simulink model "SF015A_WhlImbRejctn"  (R2013b)
settings: Solver=FixedStepDiscrete  SolverMode=SingleTasking  StartTime=0.0  StopTime=1  FixedStep=0.002  RelTol=1e-3
undefined symbols (not defined in the file): ACTIVBANDMAX_ULS_U32, ADAPVFILMAX_ULS_F32, ADJOUTPMAX_ULS_F32, ARCHGLBPRM_180OVERPI_ULS_F32, ARCHGLBPRM_2MILLISEC_SEC_F32, ARCHGLBPRM_2PI_ULS_F32, ARCHGLBPRM_FLOATZEROTHD_ULS_F32, ARCHGLBPRM_PI_ULS_F32, ARCHGLBPRM_PIOVER180_ULS_F32, ARCHGLBPRM_PIOVER2_ULS_F32, CALMINSPERCOUNT_ULS_F32, Cntr, DURATIONDISABLE_CNT_U16, FILTWHLSPDMAX_MOTRADPERSEC_F32, FRQMIN_ULS_F32, MICROSECTOMILLISEC_ULS_F32, MINSTOMILLISEC_ULS_F32, NINETY_ULS_F32, NODEBSTEP_CNT_U16, NROFDLY_CNT_U08, NtcSts1, NvmGetErrSts1, ONEHALF_ULS_F32, ONEHUNDRED_ULS_F32, ONEOVRTHREE_ULS_F32, ONEOVRTWENTY_ULS_F32, ONETHOUSAND_ULS_F32, PEAKMAX_ULS_F32, PEAKMIN_ULS_F32, PHAADJMAX_ULS_F32, PITIMESSAMPLETIME_ULS_F32, SigQlfr1, STOREDMINSPERCOUNT_ULS_F32, Sts, SysSt1, TWO_ULS_F32, TWOOVRTHREE_ULS_F32, UGRFILMAX_ULS_F32, WhlImbRejctnAdpvFac, WhlImbRejctnAutScaEna, WhlImbRejctnAutScaTar, WhlImbRejctnCurrMgnSlewPerLoop, WhlImbRejctnDcTrendFltRcvryDly, WhlImbRejctnDcTrendFltRcvryNegStep, WhlImbRejctnDcTrendFltRcvryPosStep, WhlImbRejctnDcTrendFltRcvryThd, WhlImbRejctnDcTrendTh2Tq, WhlImbRejctnDcTrendThTq, WhlImbRejctnDcTrendTi2Sec, WhlImbRejctnDcTrendTiSec, WhlImbRejctnEnaSlewPerLoop, WhlImbRejctnFctEna, WhlImbRejctnFltNtc, WhlImbRejctnFrqDiagcAmpThd, WhlImbRejctnFrqDiagcEna, WhlImbRejctnFrqDiagcFltRcvryDly, WhlImbRejctnFrqDiagcFltRcvryNegStep, WhlImbRejctnFrqDiagcFltRcvryPosStep, WhlImbRejctnFrqDiagcFltRcvryThd, WhlImbRejctnFrqDiagcThd ... (+30)
libraries: FixdToFloat x32, simulink x26, NxtrLim x25, Fil x20, NxtrAbslt x9, NxtrMath x7, NxtrMax x6, NxtrMin x4, NxtrNvM x2, FloatToFixd x2, LnrIntrpn x2, NxtrSign x1
(part 5 of 14)

== system SF015A_WhlImbRejctn/WhlImbRejctn/WhlImbRejctnPer2/Flt Recovery- WhlSpdCorr Diag/Update Fault Status ==
  Structvar : Inport
  Status : Inport  Port=2
  Bus Assignment : BusAssignment  AssignedSignals=Cntr,Sts
  Bus Selector : BusSelector  OutputSignals=Cntr,Sts,Thd,NegStep,PosStep
  Compare To Zero : simulink/Logic and Bit Operations/Compare To Zero  relop=<=  OutDataTypeStr=boolean
  Constant : Constant  Value=0  OutDataTypeStr=single
  CopyRight2 : Subsystem  Description=|  mask(Copyright Information){none=on}
      | Copyright info block.                                               
      |                                                                     
      | Place copyright information at the top of every subsystem in design.
      mask prompts: none "No parameters"
      mask help: Place copyright information at the top of every subsystem in design.
      mask Display:
      | NxtrConf = 'Nexteer Confidential';
      | 
      | sys = bdroot; %handle for the current model ("system")
      | first = get_param(sys,'Created');
      | first = first(end-3:end);  %year is last four digits
      | 
      | last = get_param(sys,'LastModifiedDate');
      | if isempty(last)
      |     last = datestr(now,'yyyy');
      | else
      |     last = last(end-3:end);
      | end
      | 
      | if strcmp(first,last)
      |     fprintf('%s -- Copyright %s Nexteer',NxtrConf,first)
      | else
      |     fprintf('%s -- %s%s- %s Nexteer',NxtrConf,char(169),first,last)
      | end
  Enumerated Constant : simulink/Sources/Enumerated Constant  OutDataTypeStr=Enum: SigQlfr1  Value=SigQlfr1.SIGQLFR_FAILD  SampleTime=inf
  Enumerated Constant1 : simulink/Sources/Enumerated Constant  OutDataTypeStr=Enum: SigQlfr1  Value=SigQlfr1.SIGQLFR_PASSD  SampleTime=inf
  If : If  IfExpression=u1
  If1 : If  NumInputs=2  IfExpression=u1  ElseIfExpressions=u2  ShowElse=off
  Merge : Merge
  Relational Operator : RelationalOperator  OutDataTypeStr=boolean
  Terminator : Terminator
  Towards Failed : Subsystem  TreatAsAtomicUnit=on
  Towards Passed : Subsystem  TreatAsAtomicUnit=on
  Update to Failed : Subsystem  TreatAsAtomicUnit=on
  Update to Passed : Subsystem  TreatAsAtomicUnit=on
  counter : Merge
  Structvar_out : Outport
  wires:
  Structvar/1 -> Bus Assignment/1, Bus Selector/1
  Status/1 -> If/1
  If/1 -> Towards Failed/Action
  If/2 -> Towards Passed/Action
  [PosStep] -> Towards Failed/1(PosStep)
  [NegStep] -> Towards Passed/1(NegStep)
  Towards Failed/1(Out1) -> counter/1
  Towards Passed/1(Out1) -> counter/2
  [Cnt] -> Towards Failed/2(Cnt)
  [Thd] -> Towards Failed/3(Thd)
  Constant/1 -> Towards Passed/3(Thd)
  counter/1 -> [Cnt_update], Compare To Zero/1, Relational Operator/1
  Relational Operator/1 -> If1/1
  If1/1 -> Update to Failed/Action
  If1/2 -> Update to Passed/Action
  Compare To Zero/1 -> If1/2
  Enumerated Constant1/1 -> Update to Passed/1(In1)
  Update to Failed/1(Out1) -> Merge/1
  Update to Passed/1(Out1) -> Merge/2
  Enumerated Constant/1 -> Update to Failed/1(In1)
  Bus Assignment/1 -> Structvar_out/1
  Merge/1 -> [Sts_update]
  Bus Selector/1 -> [Cnt]  "<Cntr>"
  Bus Selector/3 -> [Thd]  "<Thd>"
  Bus Selector/4 -> [NegStep]  "<NegStep>"
  Bus Selector/5 -> [PosStep]  "<PosStep>"
  [Cnt_update] -> Bus Assignment/2
  [Sts_update] -> Bus Assignment/3
  [Cnt] -> Towards Passed/2(Cnt)
  [Thd] -> Relational Operator/2
  Bus Selector/2 -> Terminator/1  "<Sts>"

== system SF015A_WhlImbRejctn/WhlImbRejctn/WhlImbRejctnPer2/WIR Low Speed Diagnostics/CopyRight2 ==

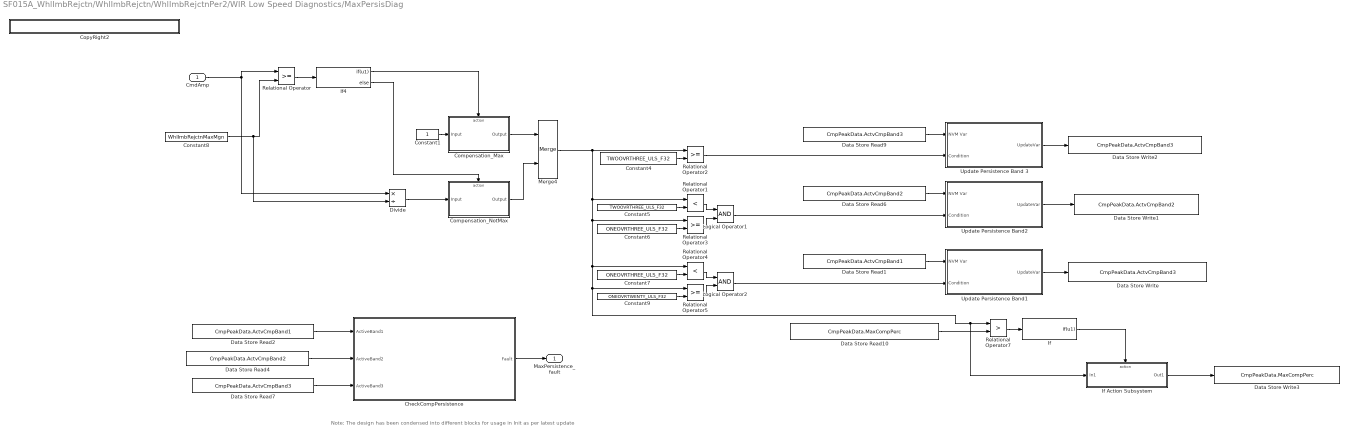
== system SF015A_WhlImbRejctn/WhlImbRejctn/WhlImbRejctnPer2/WIR Low Speed Diagnostics/MaxPersisDiag ==
  note: Note: The design has been condensed into different blocks for usage in Init as per latest update
  CmdAmp : Inport
  CheckCompPersistence : Subsystem
  Compensation_Max : Subsystem  RequirementInfo={} %GIDa_1bfe11f8_96f1_4e8d_9095_de3761426c03  TreatAsAtomicUnit=on
  Compensation_NotMax : Subsystem  RequirementInfo={} %GIDa_7b4c2964_e6f7_461b_b06a_d505129df27a  TreatAsAtomicUnit=on
  Constant1 : Constant  OutDataTypeStr=single
  Constant4 : Constant  Value=TWOOVRTHREE_ULS_F32
  Constant5 : Constant  Value=TWOOVRTHREE_ULS_F32
  Constant6 : Constant  Value=ONEOVRTHREE_ULS_F32
  Constant7 : Constant  Value=ONEOVRTHREE_ULS_F32
  Constant8 : Constant  Value=WhlImbRejctnMaxMgn
  Constant9 : Constant  Value=ONEOVRTWENTY_ULS_F32
  CopyRight2 : Subsystem  Description=|  mask(Copyright Information){none=on}
      | Copyright info block.                                               
      |                                                                     
      | Place copyright information at the top of every subsystem in design.
      mask prompts: none "No parameters"
      mask help: Place copyright information at the top of every subsystem in design.
      mask Display:
      | NxtrConf = 'Nexteer Confidential';
      | 
      | sys = bdroot; %handle for the current model ("system")
      | first = get_param(sys,'Created');
      | first = first(end-3:end);  %year is last four digits
      | 
      | last = get_param(sys,'LastModifiedDate');
      | if isempty(last)
      |     last = datestr(now,'yyyy');
      | else
      |     last = last(end-3:end);
      | end
      | 
      | if strcmp(first,last)
      |     fprintf('%s -- Copyright %s Nexteer',NxtrConf,first)
      | else
      |     fprintf('%s -- %s%s- %s Nexteer',NxtrConf,char(169),first,last)
      | end
  Data Store Read1 : DataStoreRead  Priority=1  DataStoreName=CmpPeakData  DataStoreElements=CmpPeakData.ActvCmpBand1
      settings: AttributesFormatString=Priority=%<Priority>
  Data Store Read10 : DataStoreRead  DataStoreName=CmpPeakData  DataStoreElements=CmpPeakData.MaxCompPerc
  Data Store Read2 : DataStoreRead  Priority=3  DataStoreName=CmpPeakData  DataStoreElements=CmpPeakData.ActvCmpBand1
      settings: AttributesFormatString=Priority=%<Priority>
  Data Store Read4 : DataStoreRead  Priority=3  DataStoreName=CmpPeakData  DataStoreElements=CmpPeakData.ActvCmpBand2
      settings: AttributesFormatString=Priority=%<Priority>
  Data Store Read6 : DataStoreRead  Priority=1  DataStoreName=CmpPeakData  DataStoreElements=CmpPeakData.ActvCmpBand2
      settings: AttributesFormatString=Priority=%<Priority>
  Data Store Read7 : DataStoreRead  Priority=3  DataStoreName=CmpPeakData  DataStoreElements=CmpPeakData.ActvCmpBand3
      settings: AttributesFormatString=Priority=%<Priority>
  Data Store Read9 : DataStoreRead  Priority=1  DataStoreName=CmpPeakData  DataStoreElements=CmpPeakData.ActvCmpBand3
      settings: AttributesFormatString=Priority=%<Priority>
  Data Store Write : DataStoreWrite  Priority=2  DataStoreName=CmpPeakData  DataStoreElements=CmpPeakData.ActvCmpBand3
      settings: AttributesFormatString=Priority=%<Priority>
  Data Store Write1 : DataStoreWrite  Priority=2  DataStoreName=CmpPeakData  DataStoreElements=CmpPeakData.ActvCmpBand2
      settings: AttributesFormatString=Priority=%<Priority>
  Data Store Write2 : DataStoreWrite  Priority=2  DataStoreName=CmpPeakData  DataStoreElements=CmpPeakData.ActvCmpBand3
      settings: AttributesFormatString=Priority=%<Priority>
  Data Store Write3 : DataStoreWrite  DataStoreName=CmpPeakData  DataStoreElements=CmpPeakData.MaxCompPerc
  Divide : Product  Inputs=*/
  If : If  IfExpression=u1  ShowElse=off
  If Action Subsystem : Subsystem  TreatAsAtomicUnit=on
  If4 : If  IfExpression=u1
  Logical Operator1 : Logic  AllPortsSameDT=off  OutDataTypeStr=boolean
  Logical Operator2 : Logic  AllPortsSameDT=off  OutDataTypeStr=boolean
  Merge4 : Merge
  Relational Operator{,2..3,5} (4 alike) : RelationalOperator  OutDataTypeStr=boolean
  Relational Operator1 : RelationalOperator  Operator=<  OutDataTypeStr=boolean
  Relational Operator4 : RelationalOperator  Operator=<  OutDataTypeStr=boolean
  Relational Operator7 : RelationalOperator  Operator=>  OutDataTypeStr=boolean
  Update Persistence Band 3 : Subsystem
  Update Persistence Band1 : Subsystem
  Update Persistence Band2 : Subsystem
  MaxPersistence_fault : Outport
  wires:
  CmdAmp/1 -> Relational Operator/1, Divide/1
  Constant8/1 -> Divide/2, Relational Operator/2
  Merge4/1 -> If Action Subsystem/1(In1), Relational Operator7/1, Relational Operator5/1, Relational Operator4/1, Relational Operator3/1, Relational Operator1/1, Relational Operator2/1
  Constant6/1 -> Relational Operator3/2
  Constant4/1 -> Relational Operator2/2
  Constant5/1 -> Relational Operator1/2
  Constant9/1 -> Relational Operator5/2
  Constant7/1 -> Relational Operator4/2
  Relational Operator3/1 -> Logical Operator1/2
  Relational Operator1/1 -> Logical Operator1/1
  Relational Operator4/1 -> Logical Operator2/1
  Relational Operator5/1 -> Logical Operator2/2
  Logical Operator1/1 -> Update Persistence Band2/2(Condition)
  Relational Operator7/1 -> If/1
  Data Store Read10/1 -> Relational Operator7/2
  If/1 -> If Action Subsystem/Action
  If Action Subsystem/1(Out1) -> Data Store Write3/1
  Relational Operator/1 -> If4/1
  Compensation_Max/1(Output) -> Merge4/1
  If4/1 -> Compensation_Max/Action
  Constant1/1 -> Compensation_Max/1(Input)
  Compensation_NotMax/1(Output) -> Merge4/2
  If4/2 -> Compensation_NotMax/Action
  Divide/1 -> Compensation_NotMax/1(Input)
  Data Store Read9/1 -> Update Persistence Band 3/1(NVM Var)
  Update Persistence Band 3/1(UpdateVar) -> Data Store Write2/1
  Relational Operator2/1 -> Update Persistence Band 3/2(Condition)
  Data Store Read6/1 -> Update Persistence Band2/1(NVM Var)
  Update Persistence Band2/1(UpdateVar) -> Data Store Write1/1
  Logical Operator2/1 -> Update Persistence Band1/2(Condition)
  Data Store Read1/1 -> Update Persistence Band1/1(NVM Var)
  Update Persistence Band1/1(UpdateVar) -> Data Store Write/1
  Data Store Read2/1 -> CheckCompPersistence/1(ActiveBand1)
  Data Store Read4/1 -> CheckCompPersistence/2(ActiveBand2)
  Data Store Read7/1 -> CheckCompPersistence/3(ActiveBand3)
  CheckCompPersistence/1(Fault) -> MaxPersistence_fault/1

== system SF015A_WhlImbRejctn/WhlImbRejctn/WhlImbRejctnInit1/Check NVM Data/CheckCompPersistence/CopyRight2 ==

== system SF015A_WhlImbRejctn/WhlImbRejctn/WhlImbRejctnInit1/Check NVM Data/CheckCompPersistence/NoFault ==
  Input : Inport
  Action Port : ActionPort  ActionType=else
  CopyRight2 : Subsystem  Description=|  mask(Copyright Information){none=on}
      | Copyright info block.                                               
      |                                                                     
      | Place copyright information at the top of every subsystem in design.
      mask prompts: none "No parameters"
      mask help: Place copyright information at the top of every subsystem in design.
      mask Display:
      | NxtrConf = 'Nexteer Confidential';
      | 
      | sys = bdroot; %handle for the current model ("system")
      | first = get_param(sys,'Created');
      | if(isempty(first))
      |     first = datestr(now,'yyyy');
      | else
      |     first = first(end-3:end);  %year is last four digits
      | end
      | 
      | last = get_param(sys,'LastModifiedDate');
      | if isempty(last)
      |     last = datestr(now,'yyyy');
      | else
      |     last = last(end-3:end);
      | end
      | 
      | if strcmp(first,last)
      |     fprintf('%s -- Copyright %s Nexteer',NxtrConf,first)
      | else
      |     fprintf('%s -- %s%s- %s Nexteer',NxtrConf,char(169),first,last)
      | end
  Output : Outport
  wires:
  Input/1 -> Output/1

== system SF015A_WhlImbRejctn/WhlImbRejctn/WhlImbRejctnInit1/Check NVM Data/CheckCompPersistence/Subsystem ==
  Band : Inport
  Band2 : Inport  Port=2
  Band3 : Inport  Port=3
  Action Port : ActionPort  ActionType=then
  Constant10 : Constant  Value=TWOOVRTHREE_ULS_F32
  Constant11 : Constant  Value=ONEOVRTHREE_ULS_F32
  Constant12 : Constant  Value=WhlImbRejctnMaxDurn
  Constant15 : Constant  Value=0  OutDataTypeStr=boolean
  Constant16 : Constant  OutDataTypeStr=boolean
  Constant17 : Constant  Value=STOREDMINSPERCOUNT_ULS_F32
  Constant2 : Constant  Value=CALMINSPERCOUNT_ULS_F32
  CopyRight1 : Subsystem  Description=|  mask(Copyright Information){none=on}
      | Copyright info block.                                               
      |                                                                     
      | Place copyright information at the top of every subsystem in design.
      mask prompts: none "No parameters"
      mask help: Place copyright information at the top of every subsystem in design.
      mask Display:
      | NxtrConf = 'Nexteer Confidential';
      | 
      | sys = bdroot; %handle for the current model ("system")
      | first = get_param(sys,'Created');
      | first = first(end-3:end);  %year is last four digits
      | 
      | last = get_param(sys,'LastModifiedDate');
      | if isempty(last)
      |     last = datestr(now,'yyyy');
      | else
      |     last = last(end-3:end);
      | end
      | 
      | if strcmp(first,last)
      |     fprintf('%s -- Copyright %s Nexteer',NxtrConf,first)
      | else
      |     fprintf('%s -- %s%s- %s Nexteer',NxtrConf,char(169),first,last)
      | end
  Data Type Conversion : DataTypeConversion  OutDataTypeStr=boolean
  Data Type Conversion1 : DataTypeConversion  OutDataTypeStr=boolean
  FixdToFloat_f32_u1 : FixdToFloat/FixdToFloat_f32_u32  Param1=0
  FixdToFloat_f32_u16 : FixdToFloat/FixdToFloat_f32_u16  Param1=0
  FixdToFloat_f32_u2 : FixdToFloat/FixdToFloat_f32_u32  Param1=0
  FixdToFloat_f32_u3 : FixdToFloat/FixdToFloat_f32_u32  Param1=0
  FreqDiagFault : Subsystem  RequirementInfo={} %GIDa_212db42b_1f35_4015_b5bf_9bd3bcd3665a  TreatAsAtomicUnit=on
  If5 : If  RequirementInfo={} %GIDa_d54da65b_dc62_4224_8642_661d9ee3c040  IfExpression=u1
  Merge5 : Merge
  NoFault : Subsystem  RequirementInfo={} %GIDa_c3beeaa0_bcda_4c66_a9c8_2ab73aa20fa7  TreatAsAtomicUnit=on
  Product : Product
  Product1 : Product
  Product2 : Product  RndMeth=Zero
  Product3 : Product  RndMeth=Zero
  Relational Operator6 : RelationalOperator  Operator=>  OutDataTypeStr=boolean
  Sum : Sum  Inputs=|+++
  Fault : Outport
  wires:
  Merge5/1 -> Fault/1
  Constant10/1 -> Product2/2
  Constant11/1 -> Product3/2
  Product3/1 -> Sum/3
  Product2/1 -> Sum/2
  Constant12/1 -> FixdToFloat_f32_u16/1
  Relational Operator6/1 -> If5/1
  If5/1 -> FreqDiagFault/Action
  If5/2 -> NoFault/Action
  FreqDiagFault/1(Output) -> Merge5/1
  NoFault/1(Output) -> Merge5/2
  Constant16/1 -> Data Type Conversion/1
  Constant15/1 -> Data Type Conversion1/1
  Band2/1 -> FixdToFloat_f32_u1/1
  Band3/1 -> FixdToFloat_f32_u3/1
  FixdToFloat_f32_u16/1 -> Product/1
  Data Type Conversion/1 -> FreqDiagFault/1(Input)
  Data Type Conversion1/1 -> NoFault/1(Input)
  Band/1 -> FixdToFloat_f32_u2/1
  Constant17/1 -> Product1/2
  Product/1 -> Relational Operator6/2
  Product1/1 -> Relational Operator6/1
  Sum/1 -> Product1/1
  Constant2/1 -> Product/2
  FixdToFloat_f32_u2/1 -> Sum/1
  FixdToFloat_f32_u1/1 -> Product2/1
  FixdToFloat_f32_u3/1 -> Product3/1

== system SF015A_WhlImbRejctn/WhlImbRejctn/WhlImbRejctnInit1/Check NVM Data/NvmNotVal/CopyRight2 ==

== system SF015A_WhlImbRejctn/WhlImbRejctn/WhlImbRejctnInit1/Check NVM Data/ResetNVM/CopyRight2 ==

== system SF015A_WhlImbRejctn/WhlImbRejctn/WhlImbRejctnInit1/Check NVM Data/ResetNVM1/CopyRight2 ==

== system SF015A_WhlImbRejctn/WhlImbRejctn/WhlImbRejctnPer1/Active Rejection Command /Adaptive Filter - FloatingL/CopyRight2 ==

== system SF015A_WhlImbRejctn/WhlImbRejctn/WhlImbRejctnPer1/Active Rejection Command /Adaptive Filter - FloatingR/CopyRight2 ==

== system SF015A_WhlImbRejctn/WhlImbRejctn/WhlImbRejctnPer1/Active Rejection Command /Amplitude Calculation/CopyRight2 ==

== system SF015A_WhlImbRejctn/WhlImbRejctn/WhlImbRejctnPer1/Active Rejection Command /Phase Adjust - Floating Point/Calc Filter Coefficients ==
  phase : Inport
  freq : Inport  Port=2
  CalcCoeff : Subsystem
  CalcZeroPole : Subsystem
  CopyRight2 : Subsystem  Description=|  mask(Copyright Information){none=on}
      | Copyright info block.                                               
      |                                                                     
      | Place copyright information at the top of every subsystem in design.
      mask prompts: none "No parameters"
      mask help: Place copyright information at the top of every subsystem in design.
      mask Display:
      | NxtrConf = 'Nexteer Confidential';
      | 
      | sys = bdroot; %handle for the current model ("system")
      | first = get_param(sys,'Created');
      | if(isempty(first))
      |     first = datestr(now,'yyyy');
      | else
      |     first = first(end-3:end);  %year is last four digits
      | end
      | 
      | last = get_param(sys,'LastModifiedDate');
      | if isempty(last)
      |     last = datestr(now,'yyyy');
      | else
      |     last = last(end-3:end);
      | end
      | 
      | if strcmp(first,last)
      |     fprintf('%s -- Copyright %s Nexteer',NxtrConf,first)
      | else
      |     fprintf('%s -- %s%s- %s Nexteer',NxtrConf,char(169),first,last)
      | end
  z_m : Outport
  p_k : Outport  Port=2
  b_0 : Outport  Port=3
  1/Mag : Outport  Port=4
  wires:
  CalcZeroPole/4(1/Mag at freq) -> 1/Mag/1
  freq/1 -> CalcZeroPole/2(freq)
  CalcCoeff/3(b_0) -> b_0/1
  CalcCoeff/2(p_k) -> p_k/1
  phase/1 -> CalcZeroPole/1(phase)
  CalcCoeff/1(z_m) -> z_m/1
  CalcZeroPole/3(CompGain) -> CalcCoeff/3(gain)
  CalcZeroPole/2(pole) -> CalcCoeff/2(pole)
  CalcZeroPole/1(zero) -> CalcCoeff/1(zero)

== system SF015A_WhlImbRejctn/WhlImbRejctn/WhlImbRejctnPer1/Active Rejection Command /Phase Adjust - Floating Point/CopyRight2 ==

== system SF015A_WhlImbRejctn/WhlImbRejctn/WhlImbRejctnPer1/Active Rejection Command /Phase Adjust - Floating Point/Filter 1 ==
  In1 : Inport
  z_m : Inport  Port=2
  p_k : Inport  Port=3
  b_0 : Inport  Port=4
  1/Mag : Inport  Port=5
  Add : Sum  Inputs=+-
  Add1 : Sum
  Constant1 : Constant  Value=ADJOUTPMAX_ULS_F32
  Constant2 : Constant  Value=PHAADJMAX_ULS_F32
  Constant3 : Constant  Value=PHAADJMAX_ULS_F32
  CopyRight2 : Subsystem  Description=|  mask(Copyright Information){none=on}
      | Copyright info block.                                               
      |                                                                     
      | Place copyright information at the top of every subsystem in design.
      mask prompts: none "No parameters"
      mask help: Place copyright information at the top of every subsystem in design.
      mask Display:
      | NxtrConf = 'Nexteer Confidential';
      | 
      | sys = bdroot; %handle for the current model ("system")
      | first = get_param(sys,'Created');
      | if(isempty(first))
      |     first = datestr(now,'yyyy');
      | else
      |     first = first(end-3:end);  %year is last four digits
      | end
      | 
      | last = get_param(sys,'LastModifiedDate');
      | if isempty(last)
      |     last = datestr(now,'yyyy');
      | else
      |     last = last(end-3:end);
      | end
      | 
      | if strcmp(first,last)
      |     fprintf('%s -- Copyright %s Nexteer',NxtrConf,first)
      | else
      |     fprintf('%s -- %s%s- %s Nexteer',NxtrConf,char(169),first,last)
      | end
  Data Store Read : DataStoreRead  DataStoreName=PhaAdjFil1Coeff2
  Data Store Read1 : DataStoreRead  Priority=1  DataStoreName=PhaAdjFil1Coeff1
      settings: AttributesFormatString=%<Priority 1>
  Data Store Write : DataStoreWrite  DataStoreName=PhaAdjFil1Coeff2
  Data Store Write1 : DataStoreWrite  Priority=2  DataStoreName=PhaAdjFil1Coeff1
      settings: AttributesFormatString=%<Priority 2>
  LimDyn_f1 : NxtrLim/LimDyn_f32
  LimDyn_f2 : NxtrLim/LimDyn_f32
  LimDyn_f32 : NxtrLim/LimDyn_f32
  Product : Product  RndMeth=Zero
  Product1 : Product  RndMeth=Zero
  Product2 : Product  RndMeth=Zero
  Product3 : Product  Inputs=**  RndMeth=Zero
  Unary Minus : UnaryMinus
  Unary Minus1 : UnaryMinus
  Unary Minus2 : UnaryMinus
  Out1 : Outport
  wires:
  b_0/1 -> [b_0_calc]
  [p_k_calc] -> Product2/2
  [z_m_calc] -> Product1/2
  p_k/1 -> [p_k_calc]
  z_m/1 -> [z_m_calc]
  LimDyn_f1/1 -> Data Store Write1/1, Add/1
  Product2/1 -> Add1/2
  LimDyn_f2/1 -> Data Store Write/1, Product3/1
  Add/1 -> Add1/1
  Product1/1 -> Add/2
  Data Store Read1/1 -> Product1/1  "x_n-1"
  1/Mag/1 -> Product3/2
  Data Store Read/1 -> Product2/1
  LimDyn_f32/1 -> Out1/1
  Constant1/1 -> Unary Minus/1, LimDyn_f32/3
  Unary Minus/1 -> LimDyn_f32/2
  Product3/1 -> LimDyn_f32/1
  In1/1 -> Product/1
  [b_0_calc] -> Product/2
  Constant2/1 -> Unary Minus1/1, LimDyn_f1/3
  Unary Minus1/1 -> LimDyn_f1/2
  Product/1 -> LimDyn_f1/1
  Constant3/1 -> Unary Minus2/1, LimDyn_f2/3
  Unary Minus2/1 -> LimDyn_f2/2
  Add1/1 -> LimDyn_f2/1

== system SF015A_WhlImbRejctn/WhlImbRejctn/WhlImbRejctnPer1/Active Rejection Command /Phase Adjust - Floating Point/Filter 2 ==
  In1 : Inport
  z_m : Inport  Port=2
  p_k : Inport  Port=3
  b_0 : Inport  Port=4
  1/Mag : Inport  Port=5
  Add : Sum  Inputs=+-
  Add1 : Sum
  Constant1 : Constant  Value=ADJOUTPMAX_ULS_F32
  Constant2 : Constant  Value=PHAADJMAX_ULS_F32
  Constant3 : Constant  Value=PHAADJMAX_ULS_F32
  CopyRight2 : Subsystem  Description=|  mask(Copyright Information){none=on}
      | Copyright info block.                                               
      |                                                                     
      | Place copyright information at the top of every subsystem in design.
      mask prompts: none "No parameters"
      mask help: Place copyright information at the top of every subsystem in design.
      mask Display:
      | NxtrConf = 'Nexteer Confidential';
      | 
      | sys = bdroot; %handle for the current model ("system")
      | first = get_param(sys,'Created');
      | if(isempty(first))
      |     first = datestr(now,'yyyy');
      | else
      |     first = first(end-3:end);  %year is last four digits
      | end
      | 
      | last = get_param(sys,'LastModifiedDate');
      | if isempty(last)
      |     last = datestr(now,'yyyy');
      | else
      |     last = last(end-3:end);
      | end
      | 
      | if strcmp(first,last)
      |     fprintf('%s -- Copyright %s Nexteer',NxtrConf,first)
      | else
      |     fprintf('%s -- %s%s- %s Nexteer',NxtrConf,char(169),first,last)
      | end
  Data Store Read : DataStoreRead  DataStoreName=PhaAdjFil2Coeff2
  Data Store Read1 : DataStoreRead  Priority=1  DataStoreName=PhaAdjFil2Coeff1
      settings: AttributesFormatString=%<Priority 1>
  Data Store Write : DataStoreWrite  DataStoreName=PhaAdjFil2Coeff2
  Data Store Write1 : DataStoreWrite  Priority=2  DataStoreName=PhaAdjFil2Coeff1
      settings: AttributesFormatString=%<Priority 2>
  LimDyn_f1 : NxtrLim/LimDyn_f32
  LimDyn_f2 : NxtrLim/LimDyn_f32
  LimDyn_f32 : NxtrLim/LimDyn_f32
  Product : Product  RndMeth=Zero
  Product1 : Product  RndMeth=Zero
  Product2 : Product  RndMeth=Zero
  Product3 : Product  Inputs=**  RndMeth=Zero
  Unary Minus : UnaryMinus
  Unary Minus1 : UnaryMinus
  Unary Minus2 : UnaryMinus
  Out1 : Outport
  wires:
  1/Mag/1 -> Product3/2
  Data Store Read1/1 -> Product1/1  "x_n-1"
  Product1/1 -> Add/2
  [b_0_calc] -> Product/2
  Add/1 -> Add1/1
  LimDyn_f2/1 -> Data Store Write/1, Product3/1
  Product2/1 -> Add1/2
  LimDyn_f1/1 -> Data Store Write1/1, Add/1
  z_m/1 -> [z_m_calc]
  p_k/1 -> [p_k_calc]
  [z_m_calc] -> Product1/2
  [p_k_calc] -> Product2/2
  b_0/1 -> [b_0_calc]
  Data Store Read/1 -> Product2/1
  Constant1/1 -> Unary Minus/1, LimDyn_f32/3
  Unary Minus/1 -> LimDyn_f32/2
  Product3/1 -> LimDyn_f32/1
  LimDyn_f32/1 -> Out1/1
  In1/1 -> Product/1
  Constant2/1 -> LimDyn_f1/3, Unary Minus1/1
  Unary Minus1/1 -> LimDyn_f1/2
  Product/1 -> LimDyn_f1/1
  Constant3/1 -> Unary Minus2/1, LimDyn_f2/3
  Unary Minus2/1 -> LimDyn_f2/2
  Add1/1 -> LimDyn_f2/1

== system SF015A_WhlImbRejctn/WhlImbRejctn/WhlImbRejctnPer1/Active Rejection Command /Phase Adjust - Floating Point/If Action Subsystem ==
  Pha_input : Inport
  PhaseInput : Inport  Port=2
  Action Port : ActionPort  ActionType=then
  Abslt_f32_f32 : NxtrAbslt/Abslt_f32_f32  SFunctionSpec=single y1 = Abslt_f32_f32(single u1)
      settings: AttributesFormatString=%<Name>
  Add : Sum  Inputs=-+
  Constant : Constant  Value=ARCHGLBPRM_PI_ULS_F32
  Constant1 : Constant  Value=ARCHGLBPRM_180OVERPI_ULS_F32
  CopyRight2 : Subsystem  Description=|  mask(Copyright Information){none=on}
      | Copyright info block.                                               
      |                                                                     
      | Place copyright information at the top of every subsystem in design.
      mask prompts: none "No parameters"
      mask help: Place copyright information at the top of every subsystem in design.
      mask Display:
      | NxtrConf = 'Nexteer Confidential';
      | 
      | sys = bdroot; %handle for the current model ("system")
      | first = get_param(sys,'Created');
      | if(isempty(first))
      |     first = datestr(now,'yyyy');
      | else
      |     first = first(end-3:end);  %year is last four digits
      | end
      | 
      | last = get_param(sys,'LastModifiedDate');
      | if isempty(last)
      |     last = datestr(now,'yyyy');
      | else
      |     last = last(end-3:end);
      | end
      | 
      | if strcmp(first,last)
      |     fprintf('%s -- Copyright %s Nexteer',NxtrConf,first)
      | else
      |     fprintf('%s -- %s%s- %s Nexteer',NxtrConf,char(169),first,last)
      | end
  Product : Product
  Product1 : Product
  Sign_s08_f32 : NxtrSign/Sign_s08_f32  SFunctionSpec=int8 y1 = Sign_s08_f32(single u1)
  Unary Minus : UnaryMinus
  Unary Minus1 : UnaryMinus
  Phase : Outport
  FinalPhaInput : Outport  Port=2
  wires:
  PhaseInput/1 -> Unary Minus/1
  Unary Minus/1 -> FinalPhaInput/1
  Sign_s08_f32/1 -> Unary Minus1/1
  Constant/1 -> Product/1
  Constant1/1 -> Product/2
  Product/1 -> Add/2
  Pha_input/1 -> Abslt_f32_f32/1, Sign_s08_f32/1
  Unary Minus1/1 -> Product1/1
  Add/1 -> Product1/2
  Product1/1 -> Phase/1
  Abslt_f32_f32/1 -> Add/1

== system SF015A_WhlImbRejctn/WhlImbRejctn/WhlImbRejctnPer1/Active Rejection Command /Phase Adjust - Floating Point/If Action Subsystem1 ==
  Pha_input : Inport
  PhaseInput : Inport  Port=2
  Action Port : ActionPort  ActionType=else
  CopyRight2 : Subsystem  Description=|  mask(Copyright Information){none=on}
      | Copyright info block.                                               
      |                                                                     
      | Place copyright information at the top of every subsystem in design.
      mask prompts: none "No parameters"
      mask help: Place copyright information at the top of every subsystem in design.
      mask Display:
      | NxtrConf = 'Nexteer Confidential';
      | 
      | sys = bdroot; %handle for the current model ("system")
      | first = get_param(sys,'Created');
      | if(isempty(first))
      |     first = datestr(now,'yyyy');
      | else
      |     first = first(end-3:end);  %year is last four digits
      | end
      | 
      | last = get_param(sys,'LastModifiedDate');
      | if isempty(last)
      |     last = datestr(now,'yyyy');
      | else
      |     last = last(end-3:end);
      | end
      | 
      | if strcmp(first,last)
      |     fprintf('%s -- Copyright %s Nexteer',NxtrConf,first)
      | else
      |     fprintf('%s -- %s%s- %s Nexteer',NxtrConf,char(169),first,last)
      | end
  Phase : Outport
  FinalPhaInput : Outport  Port=2
  wires:
  PhaseInput/1 -> FinalPhaInput/1
  Pha_input/1 -> Phase/1

== system SF015A_WhlImbRejctn/WhlImbRejctn/WhlImbRejctnPer1/Determine Enabled Amt/Calculate Enable1/Check_EnableDisableRange ==
  DistMagL : Inport
  DistMagR : Inport  Port=2
  DistMagEnadPrev : Inport  Port=3
  Check_for_disbale1 : Subsystem  RequirementInfo={} %GIDa_159aba51_987a_470b_b955_203c08afb92c  TreatAsAtomicUnit=on
  Check_for_disbale2 : Subsystem  RequirementInfo={} %GIDa_46258d0f_eb0e_4930_aedd_1583eb5dcf2e  TreatAsAtomicUnit=on
  Check_for_disbale3 : Subsystem  RequirementInfo={} %GIDa_a7256a8a_fc45_45b1_accf_cae14e85cdcb  TreatAsAtomicUnit=on
  Constant1 : Constant  OutDataTypeStr=boolean
  Constant12 : Constant  Value=WhlImbRejctnMgnEstimnEnaThd
  Constant15 : Constant  Value=0  OutDataTypeStr=boolean
  Constant2 : Constant  Value=0  OutDataTypeStr=boolean
  Constant5 : Constant  Value=WhlImbRejctnMgnEstimnDiThd
  CopyRight2 : Subsystem  Description=|  mask(Copyright Information){none=on}
      | Copyright info block.                                               
      |                                                                     
      | Place copyright information at the top of every subsystem in design.
      mask prompts: none "No parameters"
      mask help: Place copyright information at the top of every subsystem in design.
      mask Display:
      | NxtrConf = 'Nexteer Confidential';
      | 
      | sys = bdroot; %handle for the current model ("system")
      | first = get_param(sys,'Created');
      | first = first(end-3:end);  %year is last four digits
      | 
      | last = get_param(sys,'LastModifiedDate');
      | if isempty(last)
      |     last = datestr(now,'yyyy');
      | else
      |     last = last(end-3:end);
      | end
      | 
      | if strcmp(first,last)
      |     fprintf('%s -- Copyright %s Nexteer',NxtrConf,first)
      | else
      |     fprintf('%s -- %s%s- %s Nexteer',NxtrConf,char(169),first,last)
      | end
  Data Type Conversion1 : DataTypeConversion  OutDataTypeStr=boolean
  Data Type Conversion2 : DataTypeConversion  OutDataTypeStr=boolean
  Data Type Conversion3 : DataTypeConversion  OutDataTypeStr=boolean
  If10 : If  RequirementInfo={} %GIDa_918bc6d9_1c7e_43ab_b258_8fd3aaafebf7  NumInputs=2  IfExpression=u1  ElseIfExpressions=u2
  Logical Operator3 : Logic  AllPortsSameDT=off  OutDataTypeStr=boolean
  Logical Operator4 : Logic  Operator=OR  Inputs=3  AllPortsSameDT=off  OutDataTypeStr=boolean
  Merge6 : Merge  Inputs=3
  Relational Operator1 : RelationalOperator  Operator=>  OutDataTypeStr=boolean
  Relational Operator2 : RelationalOperator  Operator=<  OutDataTypeStr=boolean
  Relational Operator3 : RelationalOperator  Operator=>  OutDataTypeStr=boolean
  Relational Operator7 : RelationalOperator  Operator=<  OutDataTypeStr=boolean
  PrevEnabld : Outport
  wires:
  Logical Operator4/1 -> If10/2
  Merge6/1 -> PrevEnabld/1
  If10/3 -> Check_for_disbale3/Action
  Constant15/1 -> Data Type Conversion1/1
  Relational Operator2/1 -> Logical Operator3/1
  Constant5/1 -> Relational Operator2/2, Relational Operator7/2
  Relational Operator7/1 -> Logical Operator3/2
  If10/1 -> Check_for_disbale2/Action
  Logical Operator3/1 -> If10/1
  Data Type Conversion1/1 -> Check_for_disbale2/1(Input)
  DistMagR/1 -> [DistMagR]
  DistMagL/1 -> [DistMagL]
  DistMagEnadPrev/1 -> [DistMagEnadPrev]
  Check_for_disbale2/1(Output) -> Merge6/1
  [DistMagL] -> Relational Operator2/1
  [DistMagR] -> Relational Operator7/1
  [DistMagL] -> Relational Operator1/1
  [DistMagR] -> Relational Operator3/1
  Constant12/1 -> Relational Operator1/2, Relational Operator3/2
  Relational Operator1/1 -> Logical Operator4/1
  Relational Operator3/1 -> Logical Operator4/2
  [DistMagEnadPrev] -> Logical Operator4/3
  Constant1/1 -> Data Type Conversion2/1
  If10/2 -> Check_for_disbale1/Action
  Data Type Conversion2/1 -> Check_for_disbale1/1(Input)
  Check_for_disbale1/1(Output) -> Merge6/2
  Check_for_disbale3/1(Output) -> Merge6/3
  Constant2/1 -> Data Type Conversion3/1
  Data Type Conversion3/1 -> Check_for_disbale3/1(Input)

== system SF015A_WhlImbRejctn/WhlImbRejctn/WhlImbRejctnPer1/Determine Enabled Amt/Calculate Enable1/CopyRight2 ==

== system SF015A_WhlImbRejctn/WhlImbRejctn/WhlImbRejctnPer1/Determine Enabled Amt/Calculate Enable1/DistMagL ==
  note: Note: The State variable corresponding to Le and Ri are being made different
  WhlSpd : Inport
  Freq : Inport  Port=2
  Abslt_f32_f32 : NxtrAbslt/Abslt_f32_f32  SFunctionSpec=single y1 = Abslt_f32_f32(single u1)
      settings: AttributesFormatString=%<Name>
  Add1 : Sum  Inputs=+-
  Add2 : Sum
  Constant : Constant  Value=ARCHGLBPRM_PIOVER2_ULS_F32
  Constant3 : Constant  Value=WhlImbRejctnMgnEstimnFrqDelta
  Constant4 : Constant  Value=WhlImbRejctnMgnEstimnFrq
  Constant5 : Constant  Value=WhlImbRejctnMgnEstimnFrqDelta
  Constant7 : Constant  Value=WhlImbRejctnMgnEstimnFrq
  CopyRight2 : Subsystem  Description=|  mask(Copyright Information){none=on}
      | Copyright info block.                                               
      |                                                                     
      | Place copyright information at the top of every subsystem in design.
      mask prompts: none "No parameters"
      mask help: Place copyright information at the top of every subsystem in design.
      mask Display:
      | NxtrConf = 'Nexteer Confidential';
      | 
      | sys = bdroot; %handle for the current model ("system")
      | first = get_param(sys,'Created');
      | first = first(end-3:end);  %year is last four digits
      | 
      | last = get_param(sys,'LastModifiedDate');
      | if isempty(last)
      |     last = datestr(now,'yyyy');
      | else
      |     last = last(end-3:end);
      | end
      | 
      | if strcmp(first,last)
      |     fprintf('%s -- Copyright %s Nexteer',NxtrConf,first)
      | else
      |     fprintf('%s -- %s%s- %s Nexteer',NxtrConf,char(169),first,last)
      | end
  Data Store Read : DataStoreRead  DataStoreName=CmpPeakData  DataStoreElements=CmpPeakData.LePeakPrev
  Data Store Read1 : DataStoreRead  DataStoreName=CmpPeakData  DataStoreElements=CmpPeakData.LePeakPrev
  Data Store Write : DataStoreWrite  DataStoreName=CmpPeakData  DataStoreElements=CmpPeakData.LePeakPrev
  FilLpUpdOutp : Fil/FilLpUpdOutp  StVar=DistbnMgnLeLpFil
      settings: AttributesFormatString=StVar: %<StVar>
  If1 : If  RequirementInfo={} %GIDa_bbb6b281_2124_4cc1_94a0_3a6a3efe601a  IfExpression=u1
  Logical Operator : Logic  AllPortsSameDT=off  OutDataTypeStr=boolean
  Merge1 : Merge
  PeakLe : Subsystem  RequirementInfo={} %GIDa_939c926b_897c_4b71_9b35_18f6025785f3  TreatAsAtomicUnit=on
  PrevLe : Subsystem  RequirementInfo={} %GIDa_733f2386_7e78_4089_ac81_7dbfacfb5584  TreatAsAtomicUnit=on
  Product : Product  RndMeth=Zero
  Relational Operator : RelationalOperator  Operator=>  OutDataTypeStr=boolean
  Relational Operator1 : RelationalOperator  Operator=<  OutDataTypeStr=boolean
  DistMag : Outport
  CurrMag : Outport  Port=2
  wires:
  WhlSpd/1 -> Abslt_f32_f32/1
  Freq/1 -> Relational Operator/1, Relational Operator1/1
  Abslt_f32_f32/1 -> FilLpUpdOutp/1  "Temp_Var"
  FilLpUpdOutp/1 -> Product/1
  Constant/1 -> Product/2
  Product/1 -> [CurrMag], CurrMag/1
  Constant4/1 -> Add1/1
  Constant3/1 -> Add1/2
  Add1/1 -> Relational Operator/2
  Constant7/1 -> Add2/1
  Constant5/1 -> Add2/2
  Add2/1 -> Relational Operator1/2
  Relational Operator/1 -> Logical Operator/1
  Relational Operator1/1 -> Logical Operator/2
  Logical Operator/1 -> If1/1
  Merge1/1 -> Data Store Write/1, DistMag/1
  If1/1 -> PeakLe/Action
  If1/2 -> PrevLe/Action
  Data Store Read/1 -> PrevLe/1(Input)
  PrevLe/1(Output) -> Merge1/2
  PeakLe/1(Output) -> Merge1/1
  Data Store Read1/1 -> PeakLe/1(Input)
  [CurrMag] -> PeakLe/2(CurrMag)

== system SF015A_WhlImbRejctn/WhlImbRejctn/WhlImbRejctnPer1/Determine Enabled Amt/Calculate Enable1/DistMagR ==
  note: Note: The State variable corresponding to Le and Ri are being made different
  WhlSpd : Inport
  Freq : Inport  Port=2
  Abslt_f32_f32 : NxtrAbslt/Abslt_f32_f32  SFunctionSpec=single y1 = Abslt_f32_f32(single u1)
      settings: AttributesFormatString=%<Name>
  Add5 : Sum  Inputs=+-
  Add6 : Sum
  Constant11 : Constant  Value=WhlImbRejctnMgnEstimnFrqDelta
  Constant12 : Constant  Value=WhlImbRejctnMgnEstimnFrq
  Constant13 : Constant  Value=WhlImbRejctnMgnEstimnFrqDelta
  Constant14 : Constant  Value=WhlImbRejctnMgnEstimnFrq
  Constant8 : Constant  Value=ARCHGLBPRM_PIOVER2_ULS_F32
  CopyRight2 : Subsystem  Description=|  mask(Copyright Information){none=on}
      | Copyright info block.                                               
      |                                                                     
      | Place copyright information at the top of every subsystem in design.
      mask prompts: none "No parameters"
      mask help: Place copyright information at the top of every subsystem in design.
      mask Display:
      | NxtrConf = 'Nexteer Confidential';
      | 
      | sys = bdroot; %handle for the current model ("system")
      | first = get_param(sys,'Created');
      | first = first(end-3:end);  %year is last four digits
      | 
      | last = get_param(sys,'LastModifiedDate');
      | if isempty(last)
      |     last = datestr(now,'yyyy');
      | else
      |     last = last(end-3:end);
      | end
      | 
      | if strcmp(first,last)
      |     fprintf('%s -- Copyright %s Nexteer',NxtrConf,first)
      | else
      |     fprintf('%s -- %s%s- %s Nexteer',NxtrConf,char(169),first,last)
      | end
  Data Store Read1 : DataStoreRead  DataStoreName=CmpPeakData  DataStoreElements=CmpPeakData.RiPeakPrev
  Data Store Read2 : DataStoreRead  DataStoreName=CmpPeakData  DataStoreElements=CmpPeakData.RiPeakPrev
  Data Store Write : DataStoreWrite  DataStoreName=CmpPeakData  DataStoreElements=CmpPeakData.RiPeakPrev
  FilLpUpdOutp : Fil/FilLpUpdOutp  StVar=DistbnMgnRiLpFil
      settings: AttributesFormatString=StVar: %<StVar>
  If1 : If  RequirementInfo={} %GIDa_dce7b759_457d_49c0_b264_3b03eca405ed  IfExpression=u1
  Logical Operator1 : Logic  AllPortsSameDT=off  OutDataTypeStr=boolean
  Merge1 : Merge
  PeakRi : Subsystem  RequirementInfo={} %GIDa_3a74ede9_945b_43a6_9f54_5df0d5d3781d  TreatAsAtomicUnit=on
  PrevRi : Subsystem  RequirementInfo={} %GIDa_70b7393f_590a_4449_8159_0c26d2c72c5f  TreatAsAtomicUnit=on
  Product3 : Product  RndMeth=Zero
  Relational Operator2 : RelationalOperator  Operator=>  OutDataTypeStr=boolean
  Relational Operator3 : RelationalOperator  Operator=<  OutDataTypeStr=boolean
  DistMag : Outport
  CurrMag : Outport  Port=2
  wires:
  Freq/1 -> Relational Operator2/1, Relational Operator3/1
  Constant12/1 -> Add5/1
  Constant11/1 -> Add5/2
  Add5/1 -> Relational Operator2/2
  Constant14/1 -> Add6/1
  Constant13/1 -> Add6/2
  Add6/1 -> Relational Operator3/2
  Relational Operator2/1 -> Logical Operator1/1
  Relational Operator3/1 -> Logical Operator1/2
  Logical Operator1/1 -> If1/1
  If1/1 -> PeakRi/Action
  If1/2 -> PrevRi/Action
  Data Store Read2/1 -> PrevRi/1(Input)
  PrevRi/1(Output) -> Merge1/2
  PeakRi/1(Output) -> Merge1/1
  Data Store Read1/1 -> PeakRi/1(Input)
  Merge1/1 -> Data Store Write/1, DistMag/1
  [CurrMag] -> PeakRi/2(CurrMag)
  WhlSpd/1 -> Abslt_f32_f32/1
  Abslt_f32_f32/1 -> FilLpUpdOutp/1  "Temp_Var"
  FilLpUpdOutp/1 -> Product3/1
  Constant8/1 -> Product3/2
  Product3/1 -> [CurrMag], CurrMag/1

== system SF015A_WhlImbRejctn/WhlImbRejctn/WhlImbRejctnPer1/Determine Enabled Amt/Calculate Enable1/Left_AutoScale ==
  Input : Inport
  Action Port : ActionPort  ActionType=then
  CopyRight2 : Subsystem  Description=|  mask(Copyright Information){none=on}
      | Copyright info block.                                               
      |                                                                     
      | Place copyright information at the top of every subsystem in design.
      mask prompts: none "No parameters"
      mask help: Place copyright information at the top of every subsystem in design.
      mask Display:
      | NxtrConf = 'Nexteer Confidential';
      | 
      | sys = bdroot; %handle for the current model ("system")
      | first = get_param(sys,'Created');
      | if(isempty(first))
      |     first = datestr(now,'yyyy');
      | else
      |     first = first(end-3:end);  %year is last four digits
      | end
      | 
      | last = get_param(sys,'LastModifiedDate');
      | if isempty(last)
      |     last = datestr(now,'yyyy');
      | else
      |     last = last(end-3:end);
      | end
      | 
      | if strcmp(first,last)
      |     fprintf('%s -- Copyright %s Nexteer',NxtrConf,first)
      | else
      |     fprintf('%s -- %s%s- %s Nexteer',NxtrConf,char(169),first,last)
      | end
  Output : Outport
  wires:
  Input/1 -> Output/1

== system SF015A_WhlImbRejctn/WhlImbRejctn/WhlImbRejctnPer1/Determine Enabled Amt/Calculate Enable1/Left_Enable ==
  Input : Inport
  Action Port : ActionPort  ActionType=then
  CopyRight2 : Subsystem  Description=|  mask(Copyright Information){none=on}
      | Copyright info block.                                               
      |                                                                     
      | Place copyright information at the top of every subsystem in design.
      mask prompts: none "No parameters"
      mask help: Place copyright information at the top of every subsystem in design.
      mask Display:
      | NxtrConf = 'Nexteer Confidential';
      | 
      | sys = bdroot; %handle for the current model ("system")
      | first = get_param(sys,'Created');
      | if(isempty(first))
      |     first = datestr(now,'yyyy');
      | else
      |     first = first(end-3:end);  %year is last four digits
      | end
      | 
      | last = get_param(sys,'LastModifiedDate');
      | if isempty(last)
      |     last = datestr(now,'yyyy');
      | else
      |     last = last(end-3:end);
      | end
      | 
      | if strcmp(first,last)
      |     fprintf('%s -- Copyright %s Nexteer',NxtrConf,first)
      | else
      |     fprintf('%s -- %s%s- %s Nexteer',NxtrConf,char(169),first,last)
      | end
  Output : Outport
  wires:
  Input/1 -> Output/1

== system SF015A_WhlImbRejctn/WhlImbRejctn/WhlImbRejctnPer1/Determine Enabled Amt/Calculate Enable1/Left_noAutoScale ==
  Input : Inport
  Action Port : ActionPort  ActionType=else
  CopyRight2 : Subsystem  Description=|  mask(Copyright Information){none=on}
      | Copyright info block.                                               
      |                                                                     
      | Place copyright information at the top of every subsystem in design.
      mask prompts: none "No parameters"
      mask help: Place copyright information at the top of every subsystem in design.
      mask Display:
      | NxtrConf = 'Nexteer Confidential';
      | 
      | sys = bdroot; %handle for the current model ("system")
      | first = get_param(sys,'Created');
      | if(isempty(first))
      |     first = datestr(now,'yyyy');
      | else
      |     first = first(end-3:end);  %year is last four digits
      | end
      | 
      | last = get_param(sys,'LastModifiedDate');
      | if isempty(last)
      |     last = datestr(now,'yyyy');
      | else
      |     last = last(end-3:end);
      | end
      | 
      | if strcmp(first,last)
      |     fprintf('%s -- Copyright %s Nexteer',NxtrConf,first)
      | else
      |     fprintf('%s -- %s%s- %s Nexteer',NxtrConf,char(169),first,last)
      | end
  Output : Outport
  wires:
  Input/1 -> Output/1

== system SF015A_WhlImbRejctn/WhlImbRejctn/WhlImbRejctnPer1/Determine Enabled Amt/Calculate Enable1/Left_noEnable ==
  Input : Inport
  Action Port : ActionPort  ActionType=else
  CopyRight2 : Subsystem  Description=|  mask(Copyright Information){none=on}
      | Copyright info block.                                               
      |                                                                     
      | Place copyright information at the top of every subsystem in design.
      mask prompts: none "No parameters"
      mask help: Place copyright information at the top of every subsystem in design.
      mask Display:
      | NxtrConf = 'Nexteer Confidential';
      | 
      | sys = bdroot; %handle for the current model ("system")
      | first = get_param(sys,'Created');
      | if(isempty(first))
      |     first = datestr(now,'yyyy');
      | else
      |     first = first(end-3:end);  %year is last four digits
      | end
      | 
      | last = get_param(sys,'LastModifiedDate');
      | if isempty(last)
      |     last = datestr(now,'yyyy');
      | else
      |     last = last(end-3:end);
      | end
      | 
      | if strcmp(first,last)
      |     fprintf('%s -- Copyright %s Nexteer',NxtrConf,first)
      | else
      |     fprintf('%s -- %s%s- %s Nexteer',NxtrConf,char(169),first,last)
      | end
  Output : Outport
  wires:
  Input/1 -> Output/1

== system SF015A_WhlImbRejctn/WhlImbRejctn/WhlImbRejctnPer1/Determine Enabled Amt/Calculate Enable1/Right_AutoScale ==
  Input : Inport
  Action Port : ActionPort  ActionType=then
  CopyRight2 : Subsystem  Description=|  mask(Copyright Information){none=on}
      | Copyright info block.                                               
      |                                                                     
      | Place copyright information at the top of every subsystem in design.
      mask prompts: none "No parameters"
      mask help: Place copyright information at the top of every subsystem in design.
      mask Display:
      | NxtrConf = 'Nexteer Confidential';
      | 
      | sys = bdroot; %handle for the current model ("system")
      | first = get_param(sys,'Created');
      | if(isempty(first))
      |     first = datestr(now,'yyyy');
      | else
      |     first = first(end-3:end);  %year is last four digits
      | end
      | 
      | last = get_param(sys,'LastModifiedDate');
      | if isempty(last)
      |     last = datestr(now,'yyyy');
      | else
      |     last = last(end-3:end);
      | end
      | 
      | if strcmp(first,last)
      |     fprintf('%s -- Copyright %s Nexteer',NxtrConf,first)
      | else
      |     fprintf('%s -- %s%s- %s Nexteer',NxtrConf,char(169),first,last)
      | end
  Output : Outport
  wires:
  Input/1 -> Output/1

== system SF015A_WhlImbRejctn/WhlImbRejctn/WhlImbRejctnPer1/Determine Enabled Amt/Calculate Enable1/Right_Enable ==
  Input : Inport
  Action Port : ActionPort  ActionType=then
  CopyRight2 : Subsystem  Description=|  mask(Copyright Information){none=on}
      | Copyright info block.                                               
      |                                                                     
      | Place copyright information at the top of every subsystem in design.
      mask prompts: none "No parameters"
      mask help: Place copyright information at the top of every subsystem in design.
      mask Display:
      | NxtrConf = 'Nexteer Confidential';
      | 
      | sys = bdroot; %handle for the current model ("system")
      | first = get_param(sys,'Created');
      | if(isempty(first))
      |     first = datestr(now,'yyyy');
      | else
      |     first = first(end-3:end);  %year is last four digits
      | end
      | 
      | last = get_param(sys,'LastModifiedDate');
      | if isempty(last)
      |     last = datestr(now,'yyyy');
      | else
      |     last = last(end-3:end);
      | end
      | 
      | if strcmp(first,last)
      |     fprintf('%s -- Copyright %s Nexteer',NxtrConf,first)
      | else
      |     fprintf('%s -- %s%s- %s Nexteer',NxtrConf,char(169),first,last)
      | end
  Output : Outport
  wires:
  Input/1 -> Output/1
